simulink model "q11"  (R2021a)
settings: Solver=VariableStepAuto  StartTime=0.0  StopTime=100000*1e-6  RelTol=1e-3
libraries: commdigbbndpm3 x4, commutil2 x4, dspsrcs4 x4, commfilt2 x4, commchan3 x2, commsink2 x2, commrandsrc3 x2
settings Model: Creator=Fatiha  LastModifiedBy=Fatiha

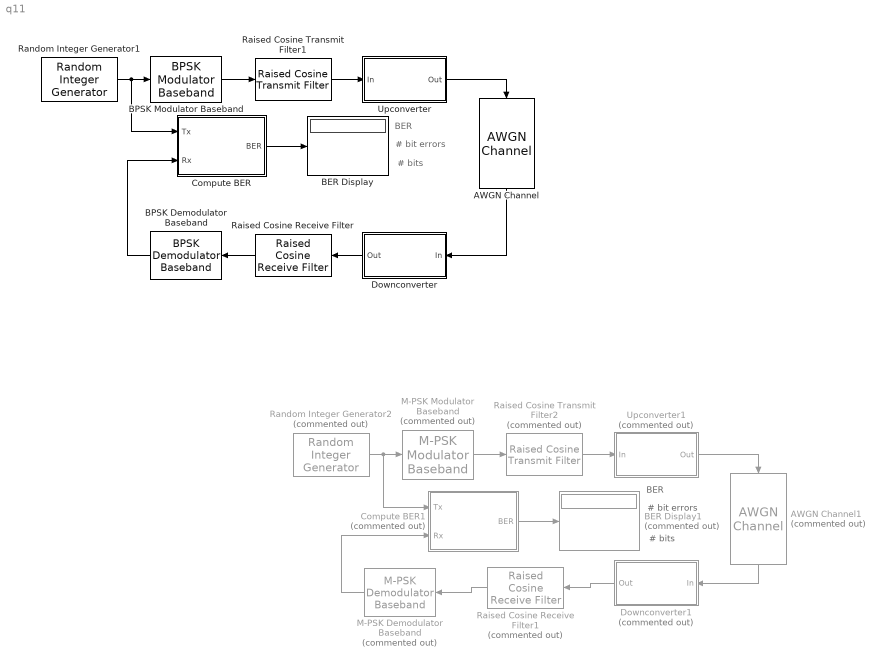
== system q11 ==
  note: BER
  note: # bit errors
  note: # bits
  note: # bit errors
  note: # bits
  note: BER
  AWGN Channel : commchan3/AWGN Channel  InputProcessing=Columns as channels (frame based)  seed=67  noiseMode="Signal to noise ratio  (Es/No)"  EbNodB=10  EsNodB=current_snr  SNRdB=10  bitsPerSym=1  Ps=1/8  Tsym=1e-6  variance=1
  AWGN Channel1 : commchan3/AWGN Channel  Commented=on  InputProcessing=Columns as channels (frame based)  seed=67  noiseMode="Signal to noise ratio  (Es/No)"  EbNodB=10  EsNodB=50  SNRdB=10  bitsPerSym=1  Ps=1/(3*8)  Tsym=1e-6  variance=1
  BER Display : Display
  BER Display1 : Display  Commented=on
  BPSK Demodulator Baseband : commdigbbndpm3/BPSK Demodulator Baseband  DecType=Hard decision  VarSource=Dialog  Variance=1  Ph=0  outDtype=Inherit via internal rule  derotateFactorWordLen=16  derotateFactorDataTypeStr=Inherit: Same word length as input  derotateFactorLastDataTypeStr=Inherit: Same word length as input
  BPSK Modulator Baseband : commdigbbndpm3/BPSK Modulator Baseband  Ph=0  outDtype=double  outWordLen=16  outUDDataType=sfix(16)  outFracLenMode=Best precision  outFracLen=15  outDataTypeStr=double  outLastDataTypeStr=double
  Compute BER : Subsystem
  Compute BER1 : Subsystem  Commented=on
  Downconverter : Subsystem
      mask Display: disp('Downconverter')
  Downconverter1 : Subsystem  Commented=on
      mask Display: disp('Downconverter')
  M-PSK Demodulator Baseband : commdigbbndpm3/M-PSK Demodulator Baseband  Commented=on  M=8  OutType=Integer  DecType=Hard decision  VarSource=Dialog  Variance=1  Dec=Gray  Mapping=[0:7]  Ph=pi/8  outDtype1=Inherit via internal rule  outDtype2=Inherit via internal rule  derotateFactorWordLen=16  derotateFactorDataTypeStr=Inherit: Same word length as input  derotateFactorLastDataTypeStr=Inherit: Same word length as input
  M-PSK Modulator Baseband : commdigbbndpm3/M-PSK Modulator Baseband  Commented=on  M=8  InType=Integer  Enc=Gray  Mapping=[0:7]  Ph=pi/8  outDtype=double  outWordLen=16  outUDDataType=sfix(16)  outFracLenMode=Best precision  outFracLen=15  outDataTypeStr=double  outLastDataTypeStr=double
  Raised Cosine Receive Filter : commfilt2/Raised Cosine Receive Filter  filtType=Square root  R=0.2  filtSpan=10  N=8  downFactor=8  downOffset=0  filterGain=1  InputProcessing=Columns as channels (frame based)  RateOptions=Enforce single-rate processing  framing=Mute  checkCoeff=off  variableName=rcRxFilt  currentFiltSpan=10  D=5  inputOffset=0  sampMode=Mute  saveAsFlag=0  rateMode=Downsampling  checkGain=Normalized  launchFVT=on  roundingMode=Floor  overflowMode=off  coeffDataTypeStr=Inherit: Same word length as input  coeffMin=[]  coeffMax=[]  coeffLastDataTypeStr=Inherit: Same word length as input  accumDataTypeStr=Inherit: Same as product output  accumLastDataTypeStr=Inherit: Same as product output  outputDataTypeStr=Inherit: Same as accumulator  outputMin=[]  outputMax=[]  outputLastDataTypeStr=Inherit: Same as accumulator
  Raised Cosine Receive Filter1 : commfilt2/Raised Cosine Receive Filter  Commented=on  filtType=Square root  R=0.2  filtSpan=10  N=8  downFactor=8  downOffset=0  filterGain=1  InputProcessing=Columns as channels (frame based)  RateOptions=Enforce single-rate processing  framing=Mute  checkCoeff=off  variableName=rcRxFilt1  currentFiltSpan=10  D=5  inputOffset=0  sampMode=Mute  saveAsFlag=0  rateMode=Downsampling  checkGain=Normalized  launchFVT=on  roundingMode=Floor  overflowMode=off  coeffDataTypeStr=Inherit: Same word length as input  coeffMin=[]  coeffMax=[]  coeffLastDataTypeStr=Inherit: Same word length as input  accumDataTypeStr=Inherit: Same as product output  accumLastDataTypeStr=Inherit: Same as product output  outputDataTypeStr=Inherit: Same as accumulator  outputMin=[]  outputMax=[]  outputLastDataTypeStr=Inherit: Same as accumulator
  Raised Cosine Transmit Filter1 : commfilt2/Raised Cosine Transmit Filter  filtType=Square root  R=0.2  filtSpan=10  N=8  filterGain=1  InputProcessing=Columns as channels (frame based)  RateOptions=Enforce single-rate processing  framing=Mute  checkCoeff=off  variableName=rcTxFilt1  checkGain=Normalized  sampMode=Mute  saveAsFlag=0  currentFiltSpan=10  D=5  launchFVT=on  roundingMode=Floor  overflowMode=off  coeffDataTypeStr=Inherit: Same word length as input  coeffMin=[]  coeffMax=[]  coeffLastDataTypeStr=Inherit: Same word length as input  outputDataTypeStr=Inherit: Same as accumulator  outputMin=[]  outputMax=[]  outputLastDataTypeStr=Inherit: Same as accumulator
  Raised Cosine Transmit Filter2 : commfilt2/Raised Cosine Transmit Filter  Commented=on  filtType=Square root  R=0.2  filtSpan=10  N=8  filterGain=1  InputProcessing=Columns as channels (frame based)  RateOptions=Enforce single-rate processing  framing=Mute  checkCoeff=off  variableName=rcTxFilt2  checkGain=Normalized  sampMode=Mute  saveAsFlag=0  currentFiltSpan=10  D=5  launchFVT=on  roundingMode=Floor  overflowMode=off  coeffDataTypeStr=Inherit: Same word length as input  coeffMin=[]  coeffMax=[]  coeffLastDataTypeStr=Inherit: Same word length as input  outputDataTypeStr=Inherit: Same as accumulator  outputMin=[]  outputMax=[]  outputLastDataTypeStr=Inherit: Same as accumulator
  Random Integer Generator1 : commrandsrc3/Random Integer Generator  SetSize=2  SeedSource=Auto  Seed=0  SampleTime=1e-6  SamplesPerFrame=100  OutputDataType=double  SimulateUsing=Interpreted execution
  Random Integer Generator2 : commrandsrc3/Random Integer Generator  Commented=on  SetSize=8  SeedSource=Auto  Seed=0  SampleTime=1e-6  SamplesPerFrame=1  OutputDataType=double  SimulateUsing=Interpreted execution
  Upconverter : Subsystem
      mask Display: disp('Upconverter')
  Upconverter1 : Subsystem  Commented=on
      mask Display: disp('Upconverter')
  wires:
  BPSK Modulator Baseband/1 -> Raised Cosine Transmit Filter1/1
  Raised Cosine Transmit Filter1/1 -> Upconverter/1(In)
  Downconverter/1(Out) -> Raised Cosine Receive Filter/1
  Raised Cosine Receive Filter/1 -> BPSK Demodulator Baseband/1
  Upconverter/1(Out) -> AWGN Channel/1
  AWGN Channel/1 -> Downconverter/1(In)
  Random Integer Generator1/1 -> Compute BER/1(Tx), BPSK Modulator Baseband/1
  Compute BER/1(BER) -> BER Display/1
  BPSK Demodulator Baseband/1 -> Compute BER/2(Rx)
  Raised Cosine Receive Filter1/1 -> M-PSK Demodulator Baseband/1
  AWGN Channel1/1 -> Downconverter1/1(In)
  Downconverter1/1(Out) -> Raised Cosine Receive Filter1/1
  Upconverter1/1(Out) -> AWGN Channel1/1
  Compute BER1/1(BER) -> BER Display1/1
  M-PSK Demodulator Baseband/1 -> Compute BER1/2(Rx)
  Random Integer Generator2/1 -> M-PSK Modulator Baseband/1, Compute BER1/1(Tx)
  Raised Cosine Transmit Filter2/1 -> Upconverter1/1(In)
  M-PSK Modulator Baseband/1 -> Raised Cosine Transmit Filter2/1

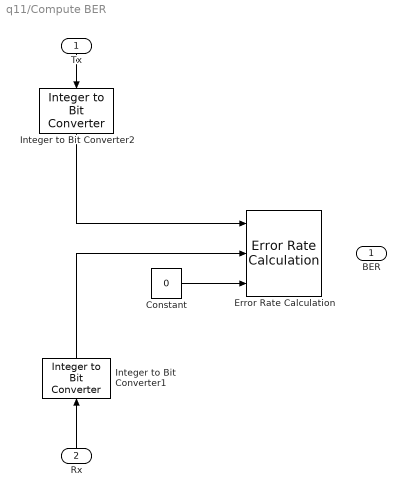
== system q11/Compute BER ==
  Tx : Inport
  Rx : Inport  Port=2
  Constant : Constant  Value=0  SampleTime=1e-4
  Error Rate Calculation : commsink2/Error Rate Calculation  N=10  st_delay=0  cp_mode=Entire frame  subframe=[]  PMode=Workspace  WsName=ErrorVec  RsMode2=on  stop=off  numErr=100  maxBits=1e6
  Integer to Bit Converter1 : commutil2/Integer to Bit Converter  nbits=1  signedInputValues=Unsigned  bitOrder=MSB first  outDtype=boolean
  Integer to Bit Converter2 : commutil2/Integer to Bit Converter  nbits=1  signedInputValues=Unsigned  bitOrder=MSB first  outDtype=boolean
  BER : Outport  VectorParamsAs1DForOutWhenUnconnected=off
  wires:
  Integer to Bit Converter2/1 -> Error Rate Calculation/1
  Integer to Bit Converter1/1 -> Error Rate Calculation/2
  Tx/1 -> Integer to Bit Converter2/1
  Rx/1 -> Integer to Bit Converter1/1
  Constant/1 -> Error Rate Calculation/3
  ? -> BER/1

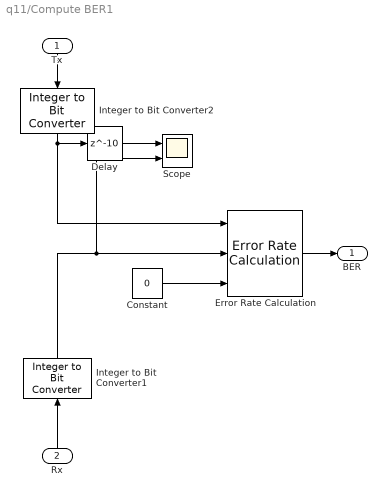
== system q11/Compute BER1 ==
  Tx : Inport
  Rx : Inport  Port=2
  Constant : Constant  Value=0  SampleTime=1e-6
  Delay : Delay  DelayLength=10
  Error Rate Calculation : commsink2/Error Rate Calculation  N=30  st_delay=0  cp_mode=Entire frame  subframe=[]  PMode=Port  WsName=ErrorVec  RsMode2=on  stop=off  numErr=100  maxBits=1e6
  Integer to Bit Converter1 : commutil2/Integer to Bit Converter  nbits=3  signedInputValues=Unsigned  bitOrder=LSB first  outDtype=boolean
  Integer to Bit Converter2 : commutil2/Integer to Bit Converter  nbits=3  signedInputValues=Unsigned  bitOrder=LSB first  outDtype=boolean
  Scope : Scope  NumInputPorts=2
  BER : Outport  VectorParamsAs1DForOutWhenUnconnected=off
  wires:
  Integer to Bit Converter2/1 -> Delay/1, Error Rate Calculation/1
  Integer to Bit Converter1/1 -> Scope/2, Error Rate Calculation/2
  Tx/1 -> Integer to Bit Converter2/1
  Error Rate Calculation/1 -> BER/1
  Rx/1 -> Integer to Bit Converter1/1
  Constant/1 -> Error Rate Calculation/3
  Delay/1 -> Scope/1

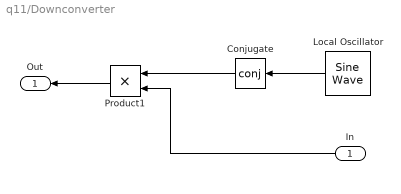
== system q11/Downconverter ==
  In : Inport
  Conjugate : Math  Operator=conj  SignedPower=on  SaturateOnIntegerOverflow=on
  Local Oscillator : dspsrcs4/Sine Wave  Amplitude=1  Frequency=2.5e6  Phase=0  SampleMode=Discrete  OutComplex=Complex  CompMethod=Trigonometric fcn  TableSize=Speed  SampleTime=(1e-6)/8  SamplesPerFrame=800  ResetState=Restart at time zero  OutputFrames=off  dataType=double  wordLen=16  udDataType=sfix(16)  fracBitsMode=Best precision  numFracBits=15  OutDataTypeStr=double  LastOutDataTypeStr=double
  Product1 : Product  RndMeth=Zero
  Out : Outport  VectorParamsAs1DForOutWhenUnconnected=off
  wires:
  Conjugate/1 -> Product1/1
  Product1/1 -> Out/1
  In/1 -> Product1/2
  Local Oscillator/1 -> Conjugate/1

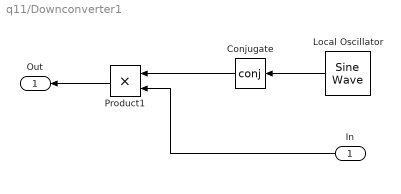
== system q11/Downconverter1 ==
  In : Inport
  Conjugate : Math  Operator=conj  SignedPower=on  SaturateOnIntegerOverflow=on
  Local Oscillator : dspsrcs4/Sine Wave  Amplitude=1  Frequency=2.5e6  Phase=0  SampleMode=Discrete  OutComplex=Complex  CompMethod=Trigonometric fcn  TableSize=Speed  SampleTime=(1e-6)/8  SamplesPerFrame=8  ResetState=Restart at time zero  OutputFrames=off  dataType=double  wordLen=16  udDataType=sfix(16)  fracBitsMode=Best precision  numFracBits=15  OutDataTypeStr=double  LastOutDataTypeStr=double
  Product1 : Product  RndMeth=Zero
  Out : Outport  VectorParamsAs1DForOutWhenUnconnected=off
  wires:
  Conjugate/1 -> Product1/1
  Product1/1 -> Out/1
  In/1 -> Product1/2
  Local Oscillator/1 -> Conjugate/1

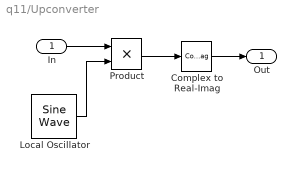
== system q11/Upconverter ==
  In : Inport
  Complex to Real-Imag : ComplexToRealImag  Output=Real
  Local Oscillator : dspsrcs4/Sine Wave  Amplitude=1  Frequency=2.5e6  Phase=0  SampleMode=Discrete  OutComplex=Complex  CompMethod=Trigonometric fcn  TableSize=Speed  SampleTime=(1e-6)/8  SamplesPerFrame=800  ResetState=Restart at time zero  OutputFrames=off  dataType=double  wordLen=16  udDataType=sfix(16)  fracBitsMode=Best precision  numFracBits=15  OutDataTypeStr=double  LastOutDataTypeStr=double
  Product : Product  RndMeth=Zero
  Out : Outport  VectorParamsAs1DForOutWhenUnconnected=off
  wires:
  Complex to Real-Imag/1 -> Out/1
  Product/1 -> Complex to Real-Imag/1
  Local Oscillator/1 -> Product/2
  In/1 -> Product/1

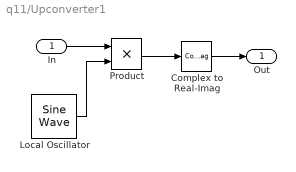
== system q11/Upconverter1 ==
  In : Inport
  Complex to Real-Imag : ComplexToRealImag  Output=Real
  Local Oscillator : dspsrcs4/Sine Wave  Amplitude=1  Frequency=2.5e6  Phase=0  SampleMode=Discrete  OutComplex=Complex  CompMethod=Trigonometric fcn  TableSize=Speed  SampleTime=(1e-6)/8  SamplesPerFrame=8  ResetState=Restart at time zero  OutputFrames=off  dataType=double  wordLen=16  udDataType=sfix(16)  fracBitsMode=Best precision  numFracBits=15  OutDataTypeStr=double  LastOutDataTypeStr=double
  Product : Product  RndMeth=Zero
  Out : Outport  VectorParamsAs1DForOutWhenUnconnected=off
  wires:
  Complex to Real-Imag/1 -> Out/1
  Product/1 -> Complex to Real-Imag/1
  Local Oscillator/1 -> Product/2
  In/1 -> Product/1
